simulink library "ParkTransformation"  (R2013a)
settings: Solver=ode45  StartTime=0.0  StopTime=10.0  RelTol=1e-3
settings Model: Creator=USER  LastModifiedBy=USER

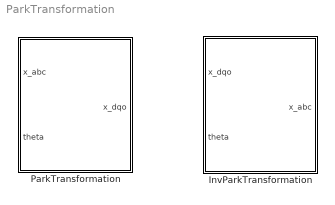
== system ParkTransformation ==
  InvParkTransformation : Subsystem
      mask help: Inverse Park Transformation
  ParkTransformation : Subsystem
      mask help: ParkTransformation

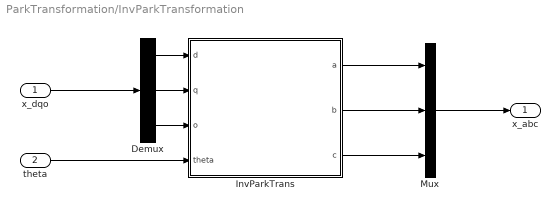
== system ParkTransformation/InvParkTransformation ==
  x_dqo : Inport
  theta : Inport  Port=2
  Demux : Demux  Outputs=3
  InvParkTrans : MATLAB Function  TreatAsAtomicUnit=on
  Mux : Mux  Inputs=3
  x_abc : Outport
  wires:
  theta/1 -> InvParkTrans/4(theta)
  x_dqo/1 -> Demux/1
  Mux/1 -> x_abc/1
  InvParkTrans/1(a) -> Mux/1
  Demux/1 -> InvParkTrans/1(d)
  Demux/2 -> InvParkTrans/2(q)
  Demux/3 -> InvParkTrans/3(o)
  InvParkTrans/2(b) -> Mux/2
  InvParkTrans/3(c) -> Mux/3

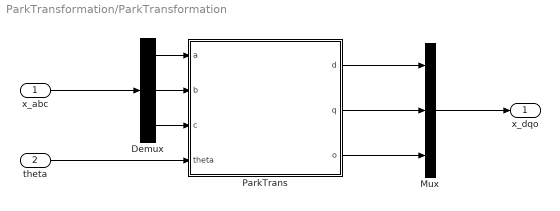
== system ParkTransformation/ParkTransformation ==
  x_abc : Inport
  theta : Inport  Port=2
  Demux : Demux  Outputs=3
  Mux : Mux  Inputs=3
  ParkTrans : MATLAB Function  TreatAsAtomicUnit=on
  x_dqo : Outport
  wires:
  theta/1 -> ParkTrans/4(theta)
  x_abc/1 -> Demux/1
  Demux/3 -> ParkTrans/3(c)
  Demux/2 -> ParkTrans/2(b)
  Demux/1 -> ParkTrans/1(a)
  Mux/1 -> x_dqo/1
  ParkTrans/3(o) -> Mux/3
  ParkTrans/2(q) -> Mux/2
  ParkTrans/1(d) -> Mux/1

== matlab function ParkTransformation/ParkTrans ==
  data: a input; d output; b input; c input; theta input; q output; o output
function [d,q,o] = fcn(a,b,c,theta)
in = [a ; b ; c];
out = sqrt(2/3)*[cos(theta), cos(theta-2*pi/3), cos(theta+2*pi/3);
                -sin(theta),-sin(theta-2*pi/3),-sin(theta+2*pi/3);
                1/sqrt(2)  , 1/sqrt(2)        ,1/sqrt(2)          ]*in;
 
q = out(1);
d = out(2);
o = out(3);

== matlab function ParkTransformation/InvParkTransformation/InvParkTrans ==
  data: a output; d input; q input; o input; b output; c output; theta input
function [a,b,c] = fcn(d,q,o,theta)
in = [d ; q ; o];
out = sqrt(2/3)*[cos(theta)      ,-sin(theta)       ,1/sqrt(2);
                cos(theta-2*pi/3),-sin(theta-2*pi/3),1/sqrt(2);
                cos(theta+2*pi/3),-sin(theta+2*pi/3),1/sqrt(2)]*in;
 
a = out(1);
b = out(2);
c = out(3);
